simulink model "PD"  (R2016b)
settings: Solver=FixedStepAuto  StartTime=0.0  StopTime=10.0  FixedStep=0.01  RelTol=1e-3
values from neighbouring files (symbols this model uses):
  den = [1 0.1313 1.109]    [UpdatedSimulinkValues-2.m]    (also in UpdatedSimulinkValuesalex1.m; part2a.m)
  num = [0.26*1.109*180/pi()]    [UpdatedSimulinkValues-2.m]    (also in UpdatedSimulinkValuesalex1.m; part2a.m)
undefined symbols (not defined in the file or in its folder): G
settings Model: Creator=Akash  LastModifiedBy=Akash
settings SolverCC: MaxConsecutiveMinStep=2

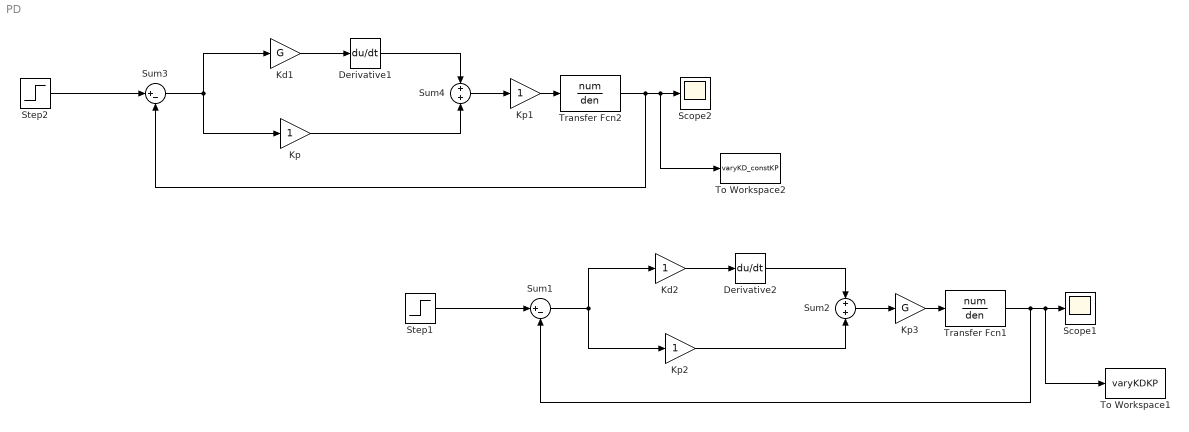
== system PD ==
  Derivative1 : Derivative
  Derivative2 : Derivative
  Kd1 : Gain  Gain=G
  Kd2 : Gain
  Kp : Gain
  Kp1 : Gain
  Kp2 : Gain
  Kp3 : Gain  Gain=G
  Scope1 : Scope
  Scope2 : Scope
  Step1 : Step  SampleTime=0
  Step2 : Step  SampleTime=0
  Sum1 : Sum  Inputs=|+-
  Sum2 : Sum
  Sum3 : Sum  Inputs=|+-
  Sum4 : Sum
  To Workspace1 : ToWorkspace  VariableName=varyKDKP  SaveFormat=Timeseries  SampleTime=-1
  To Workspace2 : ToWorkspace  VariableName=varyKD_constKP  SaveFormat=Timeseries  SampleTime=-1
  Transfer Fcn1 : TransferFcn  Numerator=num  Denominator=den
  Transfer Fcn2 : TransferFcn  Numerator=num  Denominator=den
  wires:
  Step2/1 -> Sum3/1
  Transfer Fcn2/1 -> Sum3/2, To Workspace2/1, Scope2/1
  Sum4/1 -> Kp1/1
  Derivative1/1 -> Sum4/1
  Kd1/1 -> Derivative1/1
  Sum3/1 -> Kp/1, Kd1/1
  Kp/1 -> Sum4/2
  Kp1/1 -> Transfer Fcn2/1
  Step1/1 -> Sum1/1
  Transfer Fcn1/1 -> Sum1/2, To Workspace1/1, Scope1/1
  Sum2/1 -> Kp3/1
  Derivative2/1 -> Sum2/1
  Kd2/1 -> Derivative2/1
  Sum1/1 -> Kp2/1, Kd2/1
  Kp2/1 -> Sum2/2
  Kp3/1 -> Transfer Fcn1/1
